simulink model "HW1Simulink2"  (R2024b)
settings: Solver=ode1  StartTime=0.0  StopTime=200  FixedStep=1/100  RelTol=1e-3
settings Model: Creator=yugpn  LastModifiedBy=JTerr

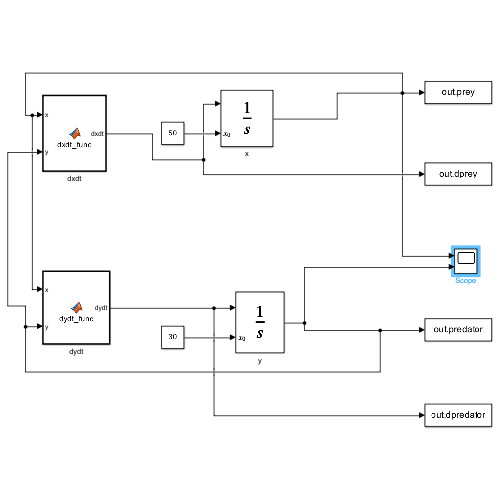
[thumbnail: Simulink's stored preview of the top-level diagram]
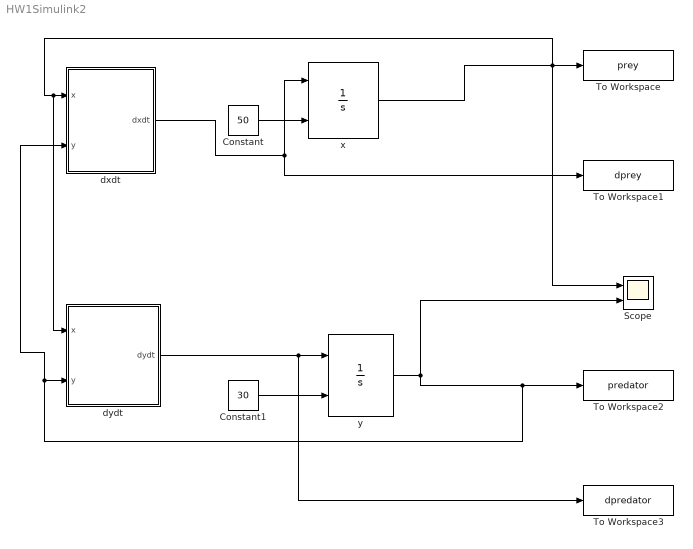
== system HW1Simulink2 ==
  Constant : Constant  Value=50
  Constant1 : Constant  Value=30
  Scope : Scope  NumInputPorts=2
  To Workspace : ToWorkspace  VariableName=prey  SampleTime=-1
      settings: Save2DSignal=2-D array (concatenate along first dimension)
  To Workspace1 : ToWorkspace  VariableName=dprey  SampleTime=-1
      settings: Save2DSignal=2-D array (concatenate along first dimension)
  To Workspace2 : ToWorkspace  VariableName=predator  SampleTime=-1
      settings: Save2DSignal=2-D array (concatenate along first dimension)
  To Workspace3 : ToWorkspace  VariableName=dpredator  SampleTime=-1
      settings: Save2DSignal=2-D array (concatenate along first dimension)
  dxdt : MATLAB Function  TreatAsAtomicUnit=on
  dydt : MATLAB Function  TreatAsAtomicUnit=on
  x : Integrator  InitialConditionSource=external  IgnoreLimit=on
  y : Integrator  InitialConditionSource=external  IgnoreLimit=on
  wires:
  Constant1/1 -> y/2
  Constant/1 -> x/2
  dxdt/1(dxdt) -> To Workspace1/1, x/1
  dydt/1(dydt) -> To Workspace3/1, y/1
  y/1 -> dxdt/2(y), dydt/2(y), To Workspace2/1, Scope/2
  x/1 -> Scope/1, To Workspace/1, dydt/1(x), dxdt/1(x)

== matlab function HW1Simulink2/dxdt ==
  data: x input; dxdt output; y input
function dxdt = dxdt_func(x, y)
    dxdt = x * (1 - x / 100) - .25 * x * y;
end

== matlab function HW1Simulink2/dydt ==
  data: x input; dydt output; y input
function dydt = dydt_func(x, y)
    dydt = -y + 0.25 * x * y;
end
